simulink model "PLL_voltagesag"  (R2025a)
settings: Solver=FixedStepAuto  StartTime=0.0  StopTime=1  FixedStep=Ts  RelTol=1e-3
values from neighbouring files (symbols this model uses):
  C_dc = 2.25    [PLLpara.m]
  Cf1 = 0.01    [PLLpara.m]
  Cf2 = 0.01    [PLLpara.m]
  dt_sag = t_c    [GFMPara.m]    (also in GFMPara_exp.m; PLLpara.m; VFMPara.m; VFMPara_exp.m)
  f_switching = 20e3    (= 20000)    [GFMPara_exp.m]    (also in PLLpara.m = 10000; VFMPara_exp.m)
  Id0 = Id    [PLLpara.m]
  Iq01 = 0    [PLLpara.m]
  Iq02 = (Ug*cos(asin((Xg*Id+Rg*Iq)/Ug))+Id*Rg-Iq*Xg)*Cf2+Iq    [PLLpara.m]
  ki_pll1 = ki    [PLLpara.m]
  kp_pll1 = kp    [PLLpara.m]
  Lc = 1e-9    (= 1e-09)    [GFMPara.m]    (also in GFMPara_exp.m; PLLpara.m; VFMPara.m; VFMPara_exp.m)
  Lf = 0.0592    [GFMPara.m]    (also in GFMPara_exp.m; PLLpara.m = 0.05; VFMPara.m = 0.05; VFMPara_exp.m = 0.05)
  Lg1 = X1    [PLLpara.m]    (also in VFMPara.m; VFMPara_exp.m)
  Lgg = Xgg    [PLLpara.m]    (also in VFMPara.m; VFMPara_exp.m)
  Rf = 1e-3    (= 0.001)    [PLLpara.m]
  Rg1 = R1    [PLLpara.m]    (also in VFMPara.m; VFMPara_exp.m = 4*R1/5)
  Rgg = Rgg    [PLLpara.m]    (also in VFMPara.m; VFMPara_exp.m)
  Sbase = 1    [GFMPara.m]    (also in GFMPara_exp.m; PLLpara.m; VFMPara.m; VFMPara_exp.m)
  t0 = t_sim_start +t_start    [PLLpara.m]    (also in VFMPara_exp.m)
  t0_sag = t_sim_start +t_start    [GFMPara.m]    (also in GFMPara_exp.m; PLLpara.m = 20; VFMPara.m; VFMPara_exp.m = 20)
  Tc = 1/f_switching    (= 5e-05)    [GFMPara_exp.m]    (also in PLLpara.m = 0.0001; VFMPara_exp.m)
  tc = t_c    [PLLpara.m]    (also in VFMPara_exp.m)
  Ts = 1/Fs    (= 1e-05)    [GFMPara.m]    (also in GFMPara_exp.m = 1e-06; PLLpara.m = 1e-06; VFMPara.m = 5e-06; VFMPara_exp.m = 1e-06)
  v_sag = Ug_fault    [GFMPara.m]    (also in GFMPara_exp.m; PLLpara.m; VFMPara.m; VFMPara_exp.m)
  Vbase = 1    [GFMPara.m]    (also in GFMPara_exp.m; PLLpara.m; VFMPara.m; VFMPara_exp.m)
  Vdc = 2.5    [PLLpara.m]
  w_i_GFL1 = 1100 *2*pi    (= 6911.5038379)    [PLLpara.m]
  w_i_GFL2 = 1100 *2*pi    (= 6911.5038379)    [PLLpara.m]
  w_pll1 = 10 *2*pi    (= 62.8318530718)    [PLLpara.m]
  w_tau1 = 1500 *2*pi    (= 9424.77796077)    [PLLpara.m]
  Wbase = 2*pi*50    (= 314.159265359)    [GFMPara.m]    (also in GFMPara_exp.m; PLLpara.m; VFMPara.m; VFMPara_exp.m)
  Zbase = Vbase/Ibase    (= 1)    [GFMPara.m]    (also in GFMPara_exp.m; PLLpara.m; VFMPara.m; VFMPara_exp.m)
undefined symbols (not defined in the file or in its folder): DiscIntNeverNeededParam, dspblkCoreblockFVToolHelper, gcbh, initial, position, postfault_SEP, sigbuilder_block, w_max, w_min, Ws
libraries: spsVoltageMeasurementLib x80, spsCurrentMeasurementLib x75, spsIdealSwitchLib x30, spsThreePhaseSeriesRLCBranchLib x21, spsControlledVoltageSourceLib x18, spsSeriesRLCBranchLib x11, powerlib_extras x10, spsHalfBridgeConverterLib x6, spsThreePhaseBreakerLib x6, spsDCVoltageSourceLib x4, spsThreePhaseFaultLib x3, cstblocks x2
(part 1 of 5)
settings Model: Creator=admin_user  LastModifiedBy=yifan
settings SolverCC: AlgebraicLoopSolver=TrustRegion
settings DataIOCC: ReturnWorkspaceOutputs=off
settings ModelReferenceCC: EnableRefExpFcnMdlSchedulingChecks=on
settings RTWCC: GPUComputeCapability=3.5  DLArmComputeVersion=19.05

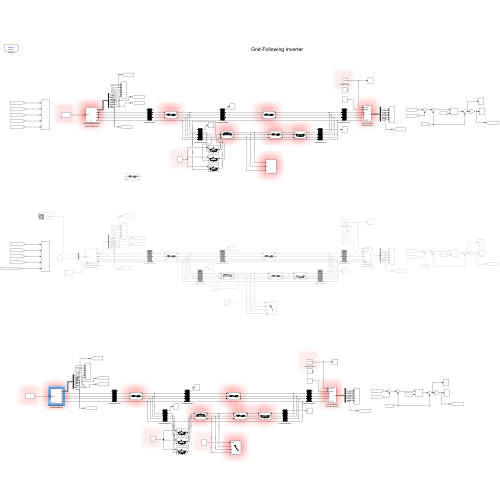
[thumbnail: Simulink's stored preview of the top-level diagram]
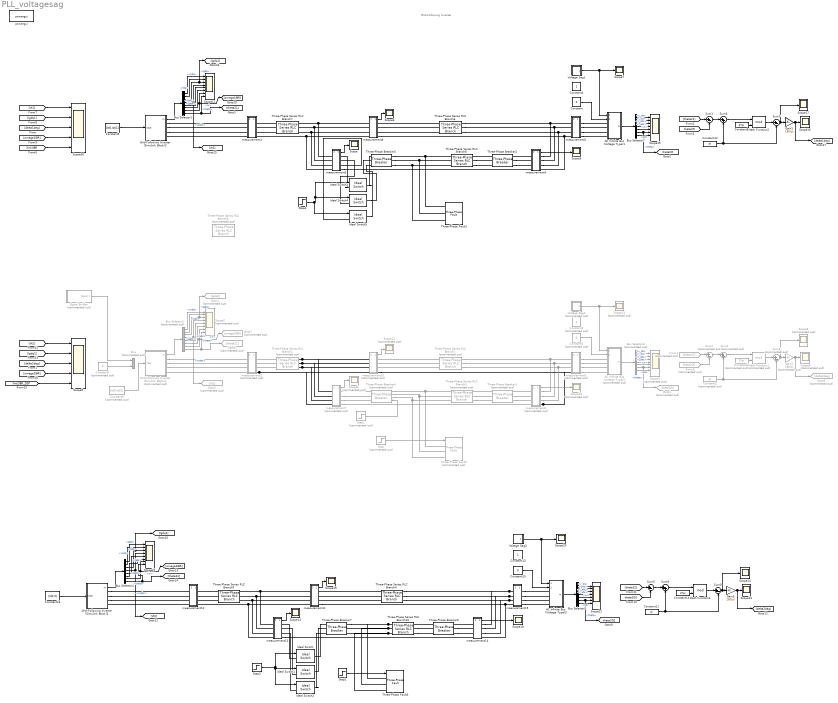
== system PLL_voltagesag ==
  note: Grid-Following Inverter
  AC Infinite Bus (Voltage Type)1 : Subsystem  AncestorBlock=|  mask{Ts=Ts, Sbase=Sbase, Vbase=Vbase, Wbase=Wbase, theta0=0, w=Wbase, R=1e-30}
      | SimplusGT/AC Infinite Bus
      | (Voltage Type)
      mask prompts: Ts "Ts (s), samping period"; Sbase "Sbase (VA), power base"; Vbase "Vbase (V), voltage base"; Wbase "Wbase (rad/s), frequency base"; theta0 "theta0 (rad), initial angle"; w "w (rad/s), frequency"; R "R (Ohm), resistance"
  AC Infinite Bus (Voltage Type)2 : Subsystem  Commented=on  AncestorBlock=|  mask{Ts=Ts, Sbase=Sbase, Vbase=Vbase, Wbase=Wbase, theta0=0, w=Wbase, R=1e-30}
      | SimplusGT/AC Infinite Bus
      | (Voltage Type)
      mask prompts: Ts "Ts (s), samping period"; Sbase "Sbase (VA), power base"; Vbase "Vbase (V), voltage base"; Wbase "Wbase (rad/s), frequency base"; theta0 "theta0 (rad), initial angle"; w "w (rad/s), frequency"; R "R (Ohm), resistance"
  AC Infinite Bus (Voltage Type)3 : Subsystem  AncestorBlock=|  mask{Ts=Ts, Sbase=Sbase, Vbase=Vbase, Wbase=Wbase, theta0=0, w=Wbase, R=1e-30}
      | SimplusGT/AC Infinite Bus
      | (Voltage Type)
      mask prompts: Ts "Ts (s), samping period"; Sbase "Sbase (VA), power base"; Vbase "Vbase (V), voltage base"; Wbase "Wbase (rad/s), frequency base"; theta0 "theta0 (rad), initial angle"; w "w (rad/s), frequency"; R "R (Ohm), resistance"
  Bus Selector1 : BusSelector  OutputSignals=vcdq,ildq,igdq,vcabc,ilabc,igabc,w,theta
  Bus Selector2 : BusSelector  Commented=on  OutputSignals=vcdq,ildq,igdq,vcabc,ilabc,igabc,w,theta
  Bus Selector3 : BusSelector  Commented=on  OutputSignals=v_dq,i_dq,v_abc,i_abc,w,theta,pq
  Bus Selector4 : BusSelector  OutputSignals=vcdq,ildq,igdq,vcabc,ilabc,igabc,w,theta
  Bus Selector5 : BusSelector  OutputSignals=v_dq,i_dq,v_abc,i_abc,w,theta,pq
  Bus Selector7 : BusSelector  OutputSignals=v_dq,i_dq,v_abc,i_abc,w,theta,pq
  Constant : Constant  Value=0
  Constant1 : Constant  Commented=on  Value=0
  Constant10 : Constant  Value=0
  Constant11 : Constant  Value=pi
  Constant12 : Constant  Value=pi
  Constant13 : Constant
  Constant14 : Constant  Value=2*pi
  Constant16 : Constant  Value=[Id0,0]
  Constant2 : Constant  Commented=on  Value=pi
  Constant3 : Constant  Commented=on
  Constant4 : Constant
  Constant5 : Constant  Value=[Id0,Iq01]
  Constant6 : Constant  Commented=on  Value=2*pi
  Constant7 : Constant  Commented=on  Value=0
  Constant8 : Constant  Commented=on  Value=[Id0,Iq02]
  Constant9 : Constant  Value=2*pi
  From4 : From  Commented=on  GotoTag=theta22
  From9 : From  Commented=on  GotoTag=theta2G2  TagVisibility=global
  Gain1 : Gain  Gain=180/pi
  Gain2 : Gain  Commented=on  Gain=180/pi
  Gain3 : Gain  Gain=180/pi
  Goto1 : Goto  Commented=on  GotoTag=theta2G2  TagVisibility=global
  Goto4 : Goto  Commented=on  GotoTag=Igdq2
  Goto5 : Goto  Commented=on  GotoTag=Vt2
  Goto6 : Goto  Commented=on  GotoTag=delta2deg
  Goto7 : Goto  Commented=on  GotoTag=omega2IBR
  Goto8 : Goto  Commented=on  GotoTag=theta22
  Grid-Following Inverter (Simulink Block)1 : Subsystem  Commented=on  AncestorBlock=|  mask{Ts=Ts, Sbase=Sbase, Vbase=Vbase, Wbase=Wbase, w_i=w_i_GFL2, w_pll=w_pll1, w_tau=w_tau1, Lf=Lf, Cf=Cf2, Lc=Lc}
      | SimplusGT/Grid-Following Inverter
      | (Simulink Block)
      mask prompts: Ts "Ts (s), sampling period"; Sbase "Sbase (VA), base power"; Vbase "Vbase (V), base voltage"; Wbase "Wbase (rad/s), base frequency"; w_i "w_i (rad/s), current-loop bandwidth"; w_pll "w_pll (rad/s), PLL bandwidth"; w_tau "w_tau (rad/s), PLL filter bandwidth"; Lf "Lf (pu), LCL filter"; Cf "Cf (pu), LCL filter"; Lc "Lc (pu), LCL filter"
  Grid-Following Inverter (Simulink Block)2 : Subsystem  AncestorBlock=|  mask{Ts=Ts, Sbase=Sbase, Vbase=Vbase, Wbase=Wbase, w_i=w_i_GFL1, w_pll=w_pll1, w_tau=w_tau1, Lf=Lf, Cf=Cf1, Lc=Lc}
      | SimplusGT/Grid-Following Inverter
      | (Simulink Block)
      mask prompts: Ts "Ts (s), sampling period"; Sbase "Sbase (VA), base power"; Vbase "Vbase (V), base voltage"; Wbase "Wbase (rad/s), base frequency"; w_i "w_i (rad/s), current-loop bandwidth"; w_pll "w_pll (rad/s), PLL bandwidth"; w_tau "w_tau (rad/s), PLL filter bandwidth"; Lf "Lf (pu), LCL filter"; Cf "Cf (pu), LCL filter"; Lc "Lc (pu), LCL filter"
  Grid-Following Inverter (Simulink Block)3 : Subsystem  AncestorBlock=|  mask{Ts=Ts, Sbase=Sbase, Vbase=Vbase, Wbase=Wbase, w_i=w_i_GFL2, w_pll=w_pll1, w_tau=w_tau1, Lf=Lf, Cf=Cf2, Lc=Lc}
      | SimplusGT/Grid-Following Inverter
      | (Simulink Block)
      mask prompts: Ts "Ts (s), sampling period"; Sbase "Sbase (VA), base power"; Vbase "Vbase (V), base voltage"; Wbase "Wbase (rad/s), base frequency"; w_i "w_i (rad/s), current-loop bandwidth"; w_pll "w_pll (rad/s), PLL bandwidth"; w_tau "w_tau (rad/s), PLL filter bandwidth"; Lf "Lf (pu), LCL filter"; Cf "Cf (pu), LCL filter"; Lc "Lc (pu), LCL filter"
  Ideal Switch{,1..5} (6 alike) : spsIdealSwitchLib/Ideal Switch  Ron=0.001  Lon=0  IC=0  Rs=5  Cs=1e-2  Measurements=off
  Math Function1 : Math  Commented=on  Operator=mod  SignedPower=on
  Math Function2 : Math  Operator=mod  SignedPower=on
  Math Function3 : Math  Operator=mod  SignedPower=on
  Mux : Mux  Commented=on  Inputs=2
  Scope{,5..7,14,16..20,23..24} (12 alike) : Scope
      Scope settings: ActiveDisplayYMinimum=-1.51038  ActiveDisplayYMaximum=1.38351
      Scope14 settings: ActiveDisplayYMinimum=-1.35141  ActiveDisplayYMaximum=1.22161
      Scope16 settings: ActiveDisplayYMinimum=-224.72735  ActiveDisplayYMaximum=224.86411  DataLoggingDecimation=10  DataLoggingVariableName=ScopeData6
      Scope17 settings: ActiveDisplayYMinimum=-3.92346  ActiveDisplayYMaximum=3.9238  DataLoggingDecimation=10  DataLoggingVariableName=log_Delta
      Scope18 settings: ActiveDisplayYMinimum=-0.66277  ActiveDisplayYMaximum=0.79991  DataLoggingVariableName=ScopeData2
      Scope19 settings: ActiveDisplayYMinimum=-3.26758  ActiveDisplayYMaximum=3.40018  DataLoggingVariableName=ScopeData3
      Scope20 settings: ActiveDisplayYMinimum=0.10658  ActiveDisplayYMaximum=1.05549  DataLoggingVariableName=ScopeData4
      Scope23 settings: ActiveDisplayYMinimum=-224.72735  ActiveDisplayYMaximum=224.86411  DataLoggingDecimation=10  DataLoggingVariableName=ScopeData7
      Scope24 settings: ActiveDisplayYMinimum=-3.92678  ActiveDisplayYMaximum=3.92693  DataLoggingDecimation=10  DataLoggingVariableName=log_Delta2
      Scope5 settings: ActiveDisplayYMinimum=-6.53351  ActiveDisplayYMaximum=8.12515  DataLoggingVariableName=ScopeData2
      Scope6 settings: ActiveDisplayYMinimum=-3.26758  ActiveDisplayYMaximum=3.40018  DataLoggingVariableName=ScopeData3
      Scope7 settings: ActiveDisplayYMinimum=0.10658  ActiveDisplayYMaximum=1.05549
  Scope{1,4,8,10,12..13} (6 alike) : Scope  Commented=on
      Scope1 settings: ActiveDisplayYMinimum=-4.56603  ActiveDisplayYMaximum=4.9186
      Scope10 settings: ActiveDisplayYMinimum=-0.66277  ActiveDisplayYMaximum=0.79991  DataLoggingVariableName=ScopeData2
      Scope12 settings: ActiveDisplayYMinimum=-3.26758  ActiveDisplayYMaximum=3.40018  DataLoggingVariableName=ScopeData3
      Scope13 settings: ActiveDisplayYMinimum=0.10658  ActiveDisplayYMaximum=1.05549  DataLoggingVariableName=ScopeData4
      Scope4 settings: ActiveDisplayYMinimum=-224.72735  ActiveDisplayYMaximum=224.86411  DataLoggingDecimation=10  DataLoggingVariableName=ScopeData7
      Scope8 settings: ActiveDisplayYMinimum=-3.92678  ActiveDisplayYMaximum=3.92693  DataLoggingDecimation=10  DataLoggingVariableName=log_Delta2
  Scope{11,15,21..22} (4 alike) : Scope  NumInputPorts=8
      Scope11 settings: ActiveDisplayYMinimum=-1.9339360338596787  ActiveDisplayYMaximum=2.6966948236171153  DataLoggingDecimation=10  DataLoggingVariableName=ScopeData3
      Scope15 settings: ActiveDisplayYMinimum=-0.125  ActiveDisplayYMaximum=1.125  DataLoggingVariableName=ScopeData5
      Scope21 settings: ActiveDisplayYMinimum=-3.066965643945478  ActiveDisplayYMaximum=2.9929362486112421  DataLoggingDecimation=10  DataLoggingVariableName=ScopeData5
      Scope22 settings: ActiveDisplayYMinimum=-0.125  ActiveDisplayYMaximum=1.125  DataLoggingVariableName=ScopeData6
  Scope2 : Scope  Commented=on  NumInputPorts=8
      settings: ActiveDisplayYMinimum=-2.4523  ActiveDisplayYMaximum=2.43362  DataLoggingDecimation=10  DataLoggingVariableName=ScopeData5
  Scope3 : Scope  Commented=on  NumInputPorts=8
      settings: ActiveDisplayYMinimum=-0.125  ActiveDisplayYMaximum=1.125  DataLoggingVariableName=ScopeData6
  Scope30 : Scope  NumInputPorts=5
      settings: TimeSpan=1  ActiveDisplayYMinimum=-2.69435  ActiveDisplayYMaximum=2.94504  DataLoggingDecimation=10
  Scope9 : Scope  NumInputPorts=5
      settings: TimeSpan=1  ActiveDisplayYMinimum=-2.46385  ActiveDisplayYMaximum=1.98854  DataLoggingDecimation=10  DataLoggingVariableName=ScopeData2
  Signal Builder : Subsystem  Tag=STV Subsys  Commented=on  LoadFcn=sigbuilder_block('load');  StartFcn=sigbuilder_block('start');  StopFcn=sigbuilder_block('stop');  ClipboardFcn=sigbuilder_block('clipboard');  mask(Sigbuilder block){tuvar=[0:10]}
      mask help: Simulink:masks:SigbuilderBlock_MD
      mask init:
      | if ~strcmp(get_param(bdroot(gcbh),'SimulationStatus'),'stopped') tuvar = sigbuilder_block('maskInit'); end
      settings: CopyFcn=sigbuilder_block('copy');  DeleteFcn=sigbuilder_block('delete');  ModelCloseFcn=sigbuilder_block('modelClose');  PreSaveFcn=sigbuilder_block('preSave');  PauseFcn=sigbuilder_block('pause');  ContinueFcn=sigbuilder_block('continue');  NameChangeFcn=sigbuilder_block('namechange');  OpenFcn=sigbuilder_block('open',[437.6 199.2 550.4 400 ]);  CloseFcn=sigbuilder_block('close');
      mask Display: plot(0, 0, 100, 100,[2, 2, 32, 32, 2], [68, 8, 8, 68, 68],[32, 2], [38, 38], [32, 19, 2],[53, 60, 44], [32, 17, 17, 2],[16, 16, 31, 31]);txt = getActiveGroup(gcbh);text(2, 100, txt,'verticalAlignment', 'top');
  Step : Step  Commented=on  Time=t0  SampleTime=0
  Step1 : Step  Commented=on  Time=t0+tc  Before=1  After=0  SampleTime=0
  Step2 : Step  Time=t0  SampleTime=0
  Step3 : Step  Time=t0+tc  Before=1  After=0  SampleTime=0
  Step4 : Step  Time=t0+tc  Before=1  After=0  SampleTime=0
  Sum{1,5,7,9} (4 alike) : Sum  Inputs=|+-
  Sum2 : Sum  Commented=on  Inputs=|+-
  Sum3 : Sum  Commented=on  Inputs=|++
  Sum4 : Sum  Commented=on  Inputs=|+-
  Sum6 : Sum  Inputs=|++
  Sum8 : Sum  Inputs=|++
  Three-Phase Series RLC Branch1 : spsThreePhaseSeriesRLCBranchLib/Three-Phase Series RLC Branch  Commented=on  LConnTagsString=A|B|C  RConnTagsString=A|B|C  BranchType=RL  Resistance=Rgg*Zbase  Inductance=Lgg*Zbase/Wbase  Capacitance=1/Wbase  Measurements=None
  Three-Phase Series RLC Branch{4,6,8,10} (4 alike) : spsThreePhaseSeriesRLCBranchLib/Three-Phase Series RLC Branch  LConnTagsString=A|B|C  RConnTagsString=A|B|C  BranchType=RL  Resistance=Rgg*Zbase  Inductance=Lgg*Zbase/Wbase  Capacitance=1/Wbase  Measurements=None
  Three-Phase Series RLC Branch2 : spsThreePhaseSeriesRLCBranchLib/Three-Phase Series RLC Branch  Commented=on  LConnTagsString=A|B|C  RConnTagsString=A|B|C  BranchType=RL  Resistance=Rg1*Zbase  Inductance=Lg1*Zbase/Wbase  Capacitance=1/Wbase  Measurements=None
  Three-Phase Series RLC Branch3 : spsThreePhaseSeriesRLCBranchLib/Three-Phase Series RLC Branch  Commented=on  LConnTagsString=A|B|C  RConnTagsString=A|B|C  BranchType=RL  Resistance=Rgg*Zbase  Inductance=Lgg*Zbase/Wbase  Capacitance=1/Wbase  Measurements=None
  Three-Phase Series RLC Branch5 : spsThreePhaseSeriesRLCBranchLib/Three-Phase Series RLC Branch  Commented=on  LConnTagsString=A|B|C  RConnTagsString=A|B|C  BranchType=RL  Resistance=1e-3 %Rgg*Zbase*(1-position)  Inductance=Lgg*Zbase/Wbase*0.1  Capacitance=1/Wbase  Measurements=None
  Three-Phase Series RLC Branch7 : spsThreePhaseSeriesRLCBranchLib/Three-Phase Series RLC Branch  LConnTagsString=A|B|C  RConnTagsString=A|B|C  BranchType=RL  Resistance=Rg1*Zbase  Inductance=Lg1*Zbase/Wbase  Capacitance=1/Wbase  Measurements=None
  Three-Phase Series RLC Branch9 : spsThreePhaseSeriesRLCBranchLib/Three-Phase Series RLC Branch  LConnTagsString=A|B|C  RConnTagsString=A|B|C  BranchType=RL  Resistance=Rg1*Zbase  Inductance=Lg1*Zbase/Wbase  Capacitance=1/Wbase  Measurements=None
  Three-Phase Breaker1 : spsThreePhaseBreakerLib/Three-Phase Breaker  Commented=on  InitialState=closed  SwitchA=on  SwitchB=on  SwitchC=on  SwitchTimes=[t0+tc]  External=off  BreakerResistance=0.01e-3  SnubberResistance=1e6  SnubberCapacitance=inf  Measurements=Breaker currents
  Three-Phase Breaker2 : spsThreePhaseBreakerLib/Three-Phase Breaker  InitialState=closed  SwitchA=on  SwitchB=on  SwitchC=on  SwitchTimes=[t0+tc]  External=off  BreakerResistance=0.01e-3  SnubberResistance=1e6  SnubberCapacitance=inf  Measurements=Breaker currents
  Three-Phase Breaker3 : spsThreePhaseBreakerLib/Three-Phase Breaker  InitialState=closed  SwitchA=on  SwitchB=on  SwitchC=on  SwitchTimes=[t0+tc]  External=off  BreakerResistance=0.1e-3  SnubberResistance=1e6  SnubberCapacitance=inf  Measurements=Breaker currents
  Three-Phase Breaker4 : spsThreePhaseBreakerLib/Three-Phase Breaker  Commented=on  InitialState=closed  SwitchA=on  SwitchB=on  SwitchC=on  SwitchTimes=[t0+tc]  External=on  BreakerResistance=0.1e-3  SnubberResistance=1e6  SnubberCapacitance=inf  Measurements=Breaker currents
  Three-Phase Breaker5 : spsThreePhaseBreakerLib/Three-Phase Breaker  InitialState=closed  SwitchA=on  SwitchB=on  SwitchC=on  SwitchTimes=[t0+tc]  External=off  BreakerResistance=0.01e-3  SnubberResistance=1e6  SnubberCapacitance=inf  Measurements=Breaker currents
  Three-Phase Breaker7 : spsThreePhaseBreakerLib/Three-Phase Breaker  InitialState=closed  SwitchA=on  SwitchB=on  SwitchC=on  SwitchTimes=[t0+tc]  External=off  BreakerResistance=0.1e-3  SnubberResistance=1e6  SnubberCapacitance=inf  Measurements=Breaker currents
  Three-Phase Fault1 : spsThreePhaseFaultLib/Three-Phase Fault  InitialStates=0  FaultA=on  FaultB=on  FaultC=on  GroundFault=on  SwitchTimes=[t0]  External=off  SwitchStatus=NaN  FaultResistance=Rf*Zbase  GroundResistance=0.01e-6  SnubberResistance=10e6  SnubberCapacitance=inf  Measurements=None
  Three-Phase Fault2 : spsThreePhaseFaultLib/Three-Phase Fault  Commented=on  InitialStates=0  FaultA=on  FaultB=on  FaultC=on  GroundFault=off  SwitchTimes=[t0]  External=on  SwitchStatus=NaN  FaultResistance=Rf*Zbase  GroundResistance=0.01e-6  SnubberResistance=10e6  SnubberCapacitance=inf  Measurements=None
  Three-Phase Fault3 : spsThreePhaseFaultLib/Three-Phase Fault  InitialStates=0  FaultA=on  FaultB=on  FaultC=on  GroundFault=on  SwitchTimes=[t0]  External=on  SwitchStatus=NaN  FaultResistance=Rf*Zbase  GroundResistance=0.01e-6  SnubberResistance=10e6  SnubberCapacitance=inf  Measurements=None
  Voltage Sag1 : Subsystem  AncestorBlock=SimplusGT/Single Pulse  mask{t0=t0_sag, dt=dt_sag, Am=v_sag}
      mask prompts: t0 "t0 (s), starting time"; dt "dt (s), pulse width"; Am "Am, pulse amplitude"
  Voltage Sag2 : Subsystem  Commented=on  AncestorBlock=SimplusGT/Single Pulse  mask{t0=t0_sag, dt=dt_sag, Am=v_sag}
      mask prompts: t0 "t0 (s), starting time"; dt "dt (s), pulse width"; Am "Am, pulse amplitude"
  Voltage Sag3 : Subsystem  AncestorBlock=SimplusGT/Single Pulse  mask{t0=t0_sag, dt=dt_sag, Am=v_sag}
      mask prompts: t0 "t0 (s), starting time"; dt "dt (s), pulse width"; Am "Am, pulse amplitude"
  measurement1 : Subsystem
      settings: PortSchema="{\"entries\":[{\"content\":{\"sides\":[{\"content\":{\"connectorIds\":[\"Out2\",\"LConn1\",\"LConn2\",\"LConn3\",\"LConn4\"]},\"type\":\"ConnectorPlacement.EquallySpacedRectSide\",\"uuid\":\"b97639c7-89ad-4c11-8fcc-ddc4f61f4533\"},{\"content\":{\"connectorIds\":[\"Out1\",\"RConn1\",\"RConn2\",\"RConn3\",\"RConn4\"],\"side\":\"RIGHT\"},\"type\":\"ConnectorPlacement.EquallySpacedRectSide\",\"uuid\":\"3b8f0759-83d7-4d3a-a5c5-bdf29e7cbe5b\"},{\"content\":{\"connectorIds\":[],\"side\":\"TOP\"},\"type\":\"ConnectorPlacement.EquallySpacedRectSide\",\"uuid\":\"1e391932-f1e1-4127-bfe0-28b7de5de667\"},{\"content\":{\"connectorIds\":[],\"side\":\"BOTTOM\"},\"type\":\"ConnectorPlacement.EquallySpacedRectSide\",\"uuid\":\"f0c236e9-048a-4270-a45f-ff2fecf0ec8b\"}]},\"type\":\"ConnectorPlacement.EquallySpacedConnector\",\"uuid\":\"002609f8-6c16-431f-ae58-b6d94c927972\"}],\"packageUris\":[\"http://schema.mathworks.com/mf0/Connector/R2020b\"],\"version\":\"1.0\"}"
  measurement10 : Subsystem  Commented=on
      settings: PortSchema="{\"entries\":[{\"content\":{\"sides\":[{\"content\":{\"connectorIds\":[\"Out2\",\"LConn1\",\"LConn2\",\"LConn3\",\"LConn4\"]},\"type\":\"ConnectorPlacement.EquallySpacedRectSide\",\"uuid\":\"b97639c7-89ad-4c11-8fcc-ddc4f61f4533\"},{\"content\":{\"connectorIds\":[\"Out1\",\"RConn1\",\"RConn2\",\"RConn3\",\"RConn4\"],\"side\":\"RIGHT\"},\"type\":\"ConnectorPlacement.EquallySpacedRectSide\",\"uuid\":\"3b8f0759-83d7-4d3a-a5c5-bdf29e7cbe5b\"},{\"content\":{\"connectorIds\":[],\"side\":\"TOP\"},\"type\":\"ConnectorPlacement.EquallySpacedRectSide\",\"uuid\":\"1e391932-f1e1-4127-bfe0-28b7de5de667\"},{\"content\":{\"connectorIds\":[],\"side\":\"BOTTOM\"},\"type\":\"ConnectorPlacement.EquallySpacedRectSide\",\"uuid\":\"f0c236e9-048a-4270-a45f-ff2fecf0ec8b\"}]},\"type\":\"ConnectorPlacement.EquallySpacedConnector\",\"uuid\":\"002609f8-6c16-431f-ae58-b6d94c927972\"}],\"packageUris\":[\"http://schema.mathworks.com/mf0/Connector/R2020b\"],\"version\":\"1.0\"}"
  measurement11 : Subsystem
      settings: PortSchema="{\"entries\":[{\"content\":{\"sides\":[{\"content\":{\"connectorIds\":[\"Out2\",\"LConn1\",\"LConn2\",\"LConn3\",\"LConn4\"]},\"type\":\"ConnectorPlacement.EquallySpacedRectSide\",\"uuid\":\"b97639c7-89ad-4c11-8fcc-ddc4f61f4533\"},{\"content\":{\"connectorIds\":[\"Out1\",\"RConn1\",\"RConn2\",\"RConn3\",\"RConn4\"],\"side\":\"RIGHT\"},\"type\":\"ConnectorPlacement.EquallySpacedRectSide\",\"uuid\":\"3b8f0759-83d7-4d3a-a5c5-bdf29e7cbe5b\"},{\"content\":{\"connectorIds\":[],\"side\":\"TOP\"},\"type\":\"ConnectorPlacement.EquallySpacedRectSide\",\"uuid\":\"1e391932-f1e1-4127-bfe0-28b7de5de667\"},{\"content\":{\"connectorIds\":[],\"side\":\"BOTTOM\"},\"type\":\"ConnectorPlacement.EquallySpacedRectSide\",\"uuid\":\"f0c236e9-048a-4270-a45f-ff2fecf0ec8b\"}]},\"type\":\"ConnectorPlacement.EquallySpacedConnector\",\"uuid\":\"002609f8-6c16-431f-ae58-b6d94c927972\"}],\"packageUris\":[\"http://schema.mathworks.com/mf0/Connector/R2020b\"],\"version\":\"1.0\"}"
  measurement12 : Subsystem
      settings: PortSchema="{\"entries\":[{\"content\":{\"sides\":[{\"content\":{\"connectorIds\":[\"Out2\",\"LConn1\",\"LConn2\",\"LConn3\",\"LConn4\"]},\"type\":\"ConnectorPlacement.EquallySpacedRectSide\",\"uuid\":\"b97639c7-89ad-4c11-8fcc-ddc4f61f4533\"},{\"content\":{\"connectorIds\":[\"Out1\",\"RConn1\",\"RConn2\",\"RConn3\",\"RConn4\"],\"side\":\"RIGHT\"},\"type\":\"ConnectorPlacement.EquallySpacedRectSide\",\"uuid\":\"3b8f0759-83d7-4d3a-a5c5-bdf29e7cbe5b\"},{\"content\":{\"connectorIds\":[],\"side\":\"TOP\"},\"type\":\"ConnectorPlacement.EquallySpacedRectSide\",\"uuid\":\"1e391932-f1e1-4127-bfe0-28b7de5de667\"},{\"content\":{\"connectorIds\":[],\"side\":\"BOTTOM\"},\"type\":\"ConnectorPlacement.EquallySpacedRectSide\",\"uuid\":\"f0c236e9-048a-4270-a45f-ff2fecf0ec8b\"}]},\"type\":\"ConnectorPlacement.EquallySpacedConnector\",\"uuid\":\"002609f8-6c16-431f-ae58-b6d94c927972\"}],\"packageUris\":[\"http://schema.mathworks.com/mf0/Connector/R2020b\"],\"version\":\"1.0\"}"
  measurement13 : Subsystem
      settings: PortSchema="{\"entries\":[{\"content\":{\"sides\":[{\"content\":{\"connectorIds\":[\"Out2\",\"LConn1\",\"LConn2\",\"LConn3\",\"LConn4\"]},\"type\":\"ConnectorPlacement.EquallySpacedRectSide\",\"uuid\":\"b97639c7-89ad-4c11-8fcc-ddc4f61f4533\"},{\"content\":{\"connectorIds\":[\"Out1\",\"RConn1\",\"RConn2\",\"RConn3\",\"RConn4\"],\"side\":\"RIGHT\"},\"type\":\"ConnectorPlacement.EquallySpacedRectSide\",\"uuid\":\"3b8f0759-83d7-4d3a-a5c5-bdf29e7cbe5b\"},{\"content\":{\"connectorIds\":[],\"side\":\"TOP\"},\"type\":\"ConnectorPlacement.EquallySpacedRectSide\",\"uuid\":\"1e391932-f1e1-4127-bfe0-28b7de5de667\"},{\"content\":{\"connectorIds\":[],\"side\":\"BOTTOM\"},\"type\":\"ConnectorPlacement.EquallySpacedRectSide\",\"uuid\":\"f0c236e9-048a-4270-a45f-ff2fecf0ec8b\"}]},\"type\":\"ConnectorPlacement.EquallySpacedConnector\",\"uuid\":\"002609f8-6c16-431f-ae58-b6d94c927972\"}],\"packageUris\":[\"http://schema.mathworks.com/mf0/Connector/R2020b\"],\"version\":\"1.0\"}"
  measurement14 : Subsystem
      settings: PortSchema="{\"entries\":[{\"content\":{\"sides\":[{\"content\":{\"connectorIds\":[\"Out2\",\"LConn1\",\"LConn2\",\"LConn3\",\"LConn4\"]},\"type\":\"ConnectorPlacement.EquallySpacedRectSide\",\"uuid\":\"b97639c7-89ad-4c11-8fcc-ddc4f61f4533\"},{\"content\":{\"connectorIds\":[\"Out1\",\"RConn1\",\"RConn2\",\"RConn3\",\"RConn4\"],\"side\":\"RIGHT\"},\"type\":\"ConnectorPlacement.EquallySpacedRectSide\",\"uuid\":\"3b8f0759-83d7-4d3a-a5c5-bdf29e7cbe5b\"},{\"content\":{\"connectorIds\":[],\"side\":\"TOP\"},\"type\":\"ConnectorPlacement.EquallySpacedRectSide\",\"uuid\":\"1e391932-f1e1-4127-bfe0-28b7de5de667\"},{\"content\":{\"connectorIds\":[],\"side\":\"BOTTOM\"},\"type\":\"ConnectorPlacement.EquallySpacedRectSide\",\"uuid\":\"f0c236e9-048a-4270-a45f-ff2fecf0ec8b\"}]},\"type\":\"ConnectorPlacement.EquallySpacedConnector\",\"uuid\":\"002609f8-6c16-431f-ae58-b6d94c927972\"}],\"packageUris\":[\"http://schema.mathworks.com/mf0/Connector/R2020b\"],\"version\":\"1.0\"}"
  measurement15 : Subsystem
      settings: PortSchema="{\"entries\":[{\"content\":{\"sides\":[{\"content\":{\"connectorIds\":[\"Out2\",\"LConn1\",\"LConn2\",\"LConn3\",\"LConn4\"]},\"type\":\"ConnectorPlacement.EquallySpacedRectSide\",\"uuid\":\"b97639c7-89ad-4c11-8fcc-ddc4f61f4533\"},{\"content\":{\"connectorIds\":[\"Out1\",\"RConn1\",\"RConn2\",\"RConn3\",\"RConn4\"],\"side\":\"RIGHT\"},\"type\":\"ConnectorPlacement.EquallySpacedRectSide\",\"uuid\":\"3b8f0759-83d7-4d3a-a5c5-bdf29e7cbe5b\"},{\"content\":{\"connectorIds\":[],\"side\":\"TOP\"},\"type\":\"ConnectorPlacement.EquallySpacedRectSide\",\"uuid\":\"1e391932-f1e1-4127-bfe0-28b7de5de667\"},{\"content\":{\"connectorIds\":[],\"side\":\"BOTTOM\"},\"type\":\"ConnectorPlacement.EquallySpacedRectSide\",\"uuid\":\"f0c236e9-048a-4270-a45f-ff2fecf0ec8b\"}]},\"type\":\"ConnectorPlacement.EquallySpacedConnector\",\"uuid\":\"002609f8-6c16-431f-ae58-b6d94c927972\"}],\"packageUris\":[\"http://schema.mathworks.com/mf0/Connector/R2020b\"],\"version\":\"1.0\"}"
  measurement2 : Subsystem  Commented=on
      settings: PortSchema="{\"entries\":[{\"content\":{\"sides\":[{\"content\":{\"connectorIds\":[\"Out2\",\"LConn1\",\"LConn2\",\"LConn3\",\"LConn4\"]},\"type\":\"ConnectorPlacement.EquallySpacedRectSide\",\"uuid\":\"b97639c7-89ad-4c11-8fcc-ddc4f61f4533\"},{\"content\":{\"connectorIds\":[\"Out1\",\"RConn1\",\"RConn2\",\"RConn3\",\"RConn4\"],\"side\":\"RIGHT\"},\"type\":\"ConnectorPlacement.EquallySpacedRectSide\",\"uuid\":\"3b8f0759-83d7-4d3a-a5c5-bdf29e7cbe5b\"},{\"content\":{\"connectorIds\":[],\"side\":\"TOP\"},\"type\":\"ConnectorPlacement.EquallySpacedRectSide\",\"uuid\":\"1e391932-f1e1-4127-bfe0-28b7de5de667\"},{\"content\":{\"connectorIds\":[],\"side\":\"BOTTOM\"},\"type\":\"ConnectorPlacement.EquallySpacedRectSide\",\"uuid\":\"f0c236e9-048a-4270-a45f-ff2fecf0ec8b\"}]},\"type\":\"ConnectorPlacement.EquallySpacedConnector\",\"uuid\":\"002609f8-6c16-431f-ae58-b6d94c927972\"}],\"packageUris\":[\"http://schema.mathworks.com/mf0/Connector/R2020b\"],\"version\":\"1.0\"}"
  measurement3 : Subsystem
      settings: PortSchema="{\"entries\":[{\"content\":{\"sides\":[{\"content\":{\"connectorIds\":[\"Out2\",\"LConn1\",\"LConn2\",\"LConn3\",\"LConn4\"]},\"type\":\"ConnectorPlacement.EquallySpacedRectSide\",\"uuid\":\"b97639c7-89ad-4c11-8fcc-ddc4f61f4533\"},{\"content\":{\"connectorIds\":[\"Out1\",\"RConn1\",\"RConn2\",\"RConn3\",\"RConn4\"],\"side\":\"RIGHT\"},\"type\":\"ConnectorPlacement.EquallySpacedRectSide\",\"uuid\":\"3b8f0759-83d7-4d3a-a5c5-bdf29e7cbe5b\"},{\"content\":{\"connectorIds\":[],\"side\":\"TOP\"},\"type\":\"ConnectorPlacement.EquallySpacedRectSide\",\"uuid\":\"1e391932-f1e1-4127-bfe0-28b7de5de667\"},{\"content\":{\"connectorIds\":[],\"side\":\"BOTTOM\"},\"type\":\"ConnectorPlacement.EquallySpacedRectSide\",\"uuid\":\"f0c236e9-048a-4270-a45f-ff2fecf0ec8b\"}]},\"type\":\"ConnectorPlacement.EquallySpacedConnector\",\"uuid\":\"002609f8-6c16-431f-ae58-b6d94c927972\"}],\"packageUris\":[\"http://schema.mathworks.com/mf0/Connector/R2020b\"],\"version\":\"1.0\"}"
  measurement4 : Subsystem
      settings: PortSchema="{\"entries\":[{\"content\":{\"sides\":[{\"content\":{\"connectorIds\":[\"Out2\",\"LConn1\",\"LConn2\",\"LConn3\",\"LConn4\"]},\"type\":\"ConnectorPlacement.EquallySpacedRectSide\",\"uuid\":\"b97639c7-89ad-4c11-8fcc-ddc4f61f4533\"},{\"content\":{\"connectorIds\":[\"Out1\",\"RConn1\",\"RConn2\",\"RConn3\",\"RConn4\"],\"side\":\"RIGHT\"},\"type\":\"ConnectorPlacement.EquallySpacedRectSide\",\"uuid\":\"3b8f0759-83d7-4d3a-a5c5-bdf29e7cbe5b\"},{\"content\":{\"connectorIds\":[],\"side\":\"TOP\"},\"type\":\"ConnectorPlacement.EquallySpacedRectSide\",\"uuid\":\"1e391932-f1e1-4127-bfe0-28b7de5de667\"},{\"content\":{\"connectorIds\":[],\"side\":\"BOTTOM\"},\"type\":\"ConnectorPlacement.EquallySpacedRectSide\",\"uuid\":\"f0c236e9-048a-4270-a45f-ff2fecf0ec8b\"}]},\"type\":\"ConnectorPlacement.EquallySpacedConnector\",\"uuid\":\"002609f8-6c16-431f-ae58-b6d94c927972\"}],\"packageUris\":[\"http://schema.mathworks.com/mf0/Connector/R2020b\"],\"version\":\"1.0\"}"
  measurement5 : Subsystem
      settings: PortSchema="{\"entries\":[{\"content\":{\"sides\":[{\"content\":{\"connectorIds\":[\"Out2\",\"LConn1\",\"LConn2\",\"LConn3\",\"LConn4\"]},\"type\":\"ConnectorPlacement.EquallySpacedRectSide\",\"uuid\":\"b97639c7-89ad-4c11-8fcc-ddc4f61f4533\"},{\"content\":{\"connectorIds\":[\"Out1\",\"RConn1\",\"RConn2\",\"RConn3\",\"RConn4\"],\"side\":\"RIGHT\"},\"type\":\"ConnectorPlacement.EquallySpacedRectSide\",\"uuid\":\"3b8f0759-83d7-4d3a-a5c5-bdf29e7cbe5b\"},{\"content\":{\"connectorIds\":[],\"side\":\"TOP\"},\"type\":\"ConnectorPlacement.EquallySpacedRectSide\",\"uuid\":\"1e391932-f1e1-4127-bfe0-28b7de5de667\"},{\"content\":{\"connectorIds\":[],\"side\":\"BOTTOM\"},\"type\":\"ConnectorPlacement.EquallySpacedRectSide\",\"uuid\":\"f0c236e9-048a-4270-a45f-ff2fecf0ec8b\"}]},\"type\":\"ConnectorPlacement.EquallySpacedConnector\",\"uuid\":\"002609f8-6c16-431f-ae58-b6d94c927972\"}],\"packageUris\":[\"http://schema.mathworks.com/mf0/Connector/R2020b\"],\"version\":\"1.0\"}"
  measurement6 : Subsystem
      settings: PortSchema="{\"entries\":[{\"content\":{\"sides\":[{\"content\":{\"connectorIds\":[\"Out2\",\"LConn1\",\"LConn2\",\"LConn3\",\"LConn4\"]},\"type\":\"ConnectorPlacement.EquallySpacedRectSide\",\"uuid\":\"b97639c7-89ad-4c11-8fcc-ddc4f61f4533\"},{\"content\":{\"connectorIds\":[\"Out1\",\"RConn1\",\"RConn2\",\"RConn3\",\"RConn4\"],\"side\":\"RIGHT\"},\"type\":\"ConnectorPlacement.EquallySpacedRectSide\",\"uuid\":\"3b8f0759-83d7-4d3a-a5c5-bdf29e7cbe5b\"},{\"content\":{\"connectorIds\":[],\"side\":\"TOP\"},\"type\":\"ConnectorPlacement.EquallySpacedRectSide\",\"uuid\":\"1e391932-f1e1-4127-bfe0-28b7de5de667\"},{\"content\":{\"connectorIds\":[],\"side\":\"BOTTOM\"},\"type\":\"ConnectorPlacement.EquallySpacedRectSide\",\"uuid\":\"f0c236e9-048a-4270-a45f-ff2fecf0ec8b\"}]},\"type\":\"ConnectorPlacement.EquallySpacedConnector\",\"uuid\":\"002609f8-6c16-431f-ae58-b6d94c927972\"}],\"packageUris\":[\"http://schema.mathworks.com/mf0/Connector/R2020b\"],\"version\":\"1.0\"}"
  measurement7 : Subsystem  Commented=on
      settings: PortSchema="{\"entries\":[{\"content\":{\"sides\":[{\"content\":{\"connectorIds\":[\"Out2\",\"LConn1\",\"LConn2\",\"LConn3\",\"LConn4\"]},\"type\":\"ConnectorPlacement.EquallySpacedRectSide\",\"uuid\":\"b97639c7-89ad-4c11-8fcc-ddc4f61f4533\"},{\"content\":{\"connectorIds\":[\"Out1\",\"RConn1\",\"RConn2\",\"RConn3\",\"RConn4\"],\"side\":\"RIGHT\"},\"type\":\"ConnectorPlacement.EquallySpacedRectSide\",\"uuid\":\"3b8f0759-83d7-4d3a-a5c5-bdf29e7cbe5b\"},{\"content\":{\"connectorIds\":[],\"side\":\"TOP\"},\"type\":\"ConnectorPlacement.EquallySpacedRectSide\",\"uuid\":\"1e391932-f1e1-4127-bfe0-28b7de5de667\"},{\"content\":{\"connectorIds\":[],\"side\":\"BOTTOM\"},\"type\":\"ConnectorPlacement.EquallySpacedRectSide\",\"uuid\":\"f0c236e9-048a-4270-a45f-ff2fecf0ec8b\"}]},\"type\":\"ConnectorPlacement.EquallySpacedConnector\",\"uuid\":\"002609f8-6c16-431f-ae58-b6d94c927972\"}],\"packageUris\":[\"http://schema.mathworks.com/mf0/Connector/R2020b\"],\"version\":\"1.0\"}"
  measurement8 : Subsystem  Commented=on
      settings: PortSchema="{\"entries\":[{\"content\":{\"sides\":[{\"content\":{\"connectorIds\":[\"Out2\",\"LConn1\",\"LConn2\",\"LConn3\",\"LConn4\"]},\"type\":\"ConnectorPlacement.EquallySpacedRectSide\",\"uuid\":\"b97639c7-89ad-4c11-8fcc-ddc4f61f4533\"},{\"content\":{\"connectorIds\":[\"Out1\",\"RConn1\",\"RConn2\",\"RConn3\",\"RConn4\"],\"side\":\"RIGHT\"},\"type\":\"ConnectorPlacement.EquallySpacedRectSide\",\"uuid\":\"3b8f0759-83d7-4d3a-a5c5-bdf29e7cbe5b\"},{\"content\":{\"connectorIds\":[],\"side\":\"TOP\"},\"type\":\"ConnectorPlacement.EquallySpacedRectSide\",\"uuid\":\"1e391932-f1e1-4127-bfe0-28b7de5de667\"},{\"content\":{\"connectorIds\":[],\"side\":\"BOTTOM\"},\"type\":\"ConnectorPlacement.EquallySpacedRectSide\",\"uuid\":\"f0c236e9-048a-4270-a45f-ff2fecf0ec8b\"}]},\"type\":\"ConnectorPlacement.EquallySpacedConnector\",\"uuid\":\"002609f8-6c16-431f-ae58-b6d94c927972\"}],\"packageUris\":[\"http://schema.mathworks.com/mf0/Connector/R2020b\"],\"version\":\"1.0\"}"
  measurement9 : Subsystem  Commented=on
      settings: PortSchema="{\"entries\":[{\"content\":{\"sides\":[{\"content\":{\"connectorIds\":[\"Out2\",\"LConn1\",\"LConn2\",\"LConn3\",\"LConn4\"]},\"type\":\"ConnectorPlacement.EquallySpacedRectSide\",\"uuid\":\"b97639c7-89ad-4c11-8fcc-ddc4f61f4533\"},{\"content\":{\"connectorIds\":[\"Out1\",\"RConn1\",\"RConn2\",\"RConn3\",\"RConn4\"],\"side\":\"RIGHT\"},\"type\":\"ConnectorPlacement.EquallySpacedRectSide\",\"uuid\":\"3b8f0759-83d7-4d3a-a5c5-bdf29e7cbe5b\"},{\"content\":{\"connectorIds\":[],\"side\":\"TOP\"},\"type\":\"ConnectorPlacement.EquallySpacedRectSide\",\"uuid\":\"1e391932-f1e1-4127-bfe0-28b7de5de667\"},{\"content\":{\"connectorIds\":[],\"side\":\"BOTTOM\"},\"type\":\"ConnectorPlacement.EquallySpacedRectSide\",\"uuid\":\"f0c236e9-048a-4270-a45f-ff2fecf0ec8b\"}]},\"type\":\"ConnectorPlacement.EquallySpacedConnector\",\"uuid\":\"002609f8-6c16-431f-ae58-b6d94c927972\"}],\"packageUris\":[\"http://schema.mathworks.com/mf0/Connector/R2020b\"],\"version\":\"1.0\"}"
  powergui : spspowerguiLib/powergui  Priority=1  SimulationMode=Discrete  SampleTime=Ts  frequency=60  Iterations=50  frequencyindice=0  Pbase=100e6  ErrMax=1e-4  UnitsV=kV  UnitsW=MW  buscounter=0  FunctionMessages=off  echomessages=off  EnableUseOfTLC=off  CurrentSourceSwitches=off  DisableSnubberDevices=off  DisableRonSwitches=off  DisableVfSwitches=off  DisplayEquations=off  AutomaticDiscreteSolvers=off  SolverType=Tustin/Backward Euler (TBE)  Interpol=off  ExternalGateDelay=off  methode=off  Ts=100  x0status=blocks  SPID=on  SwTol=0  HookPort=off  NonlinearTolerance=1e-4  nMaxIteration=100  ContinueOnMaxIteration=off  RestoreLinks=warning  ResistiveCurrentMeasurement=off  Frange=[0:2:500]  Ylog=off  Xlog=on  ShowGrid=off  save=off  variable=ZData  structure=0  ZoomFFT=off  StartTime=0.0  cycles=1  DisplayStyle=1  fundamental=60  FreqAxis=off  MaxFrequency=1000  frequencyindicesteady=1  RmsSteady=1  display=off
  tag scope: theta2G2=global, theta2G=global
  wires:
  [theta21] -> Sum1/1
  Bus Selector1/7 -> [omega1IBR], Scope11/7  "<w>"
  Grid-Following Inverter (Simulink Block)2/1(m) -> Bus Selector1/1
  Bus Selector1/2 -> Scope11/2  "<ildq>"
  Bus Selector1/5 -> Scope11/5  "<ilabc>"
  Constant12/1 -> Sum6/2, Sum7/2
  Sum1/1 -> Sum6/1
  Bus Selector7/3 -> Scope15/3  "<v_abc>"
  AC Infinite Bus (Voltage Type)1/1(m) -> Bus Selector7/1
  Constant9/1 -> Math Function2/2
  [theta2G] -> Sum1/2
  Gain1/1 -> [delta1deg], Scope16/1
  Bus Selector1/6 -> Scope11/6  "<igabc>"
  Bus Selector7/4 -> Scope15/4  "<i_abc>"
  Bus Selector7/5 -> Scope15/5  "<w>"
  Sum7/1 -> Scope17/1, Gain1/1
  Sum6/1 -> Math Function2/1
  Math Function2/1 -> Sum7/1
  Bus Selector7/7 -> Scope15/7  "<pq>"
  Bus Selector7/6 -> [theta2G], Scope15/6  "<theta>"
  Bus Selector7/1 -> Scope15/1  "<v_dq>"
  Bus Selector1/4 -> [Vt1], Scope11/4  "<vcabc>"
  Bus Selector1/1 -> Scope11/1  "<vcdq>"
  Bus Selector1/3 -> [Igdq1], Scope11/3  "<igdq>"
  Constant/1 -> AC Infinite Bus (Voltage Type)1/2(Phase)
  Bus Selector7/2 -> Scope15/2  "<i_dq>"
  Bus Selector1/8 -> [theta21], Scope11/8  "<theta>"
  [Vt1] -> Scope30/1
  [Igdq1] -> Scope30/2
  [Xint1IBR] -> Scope30/5
  [delta1deg] -> Scope30/3
  [omega1IBR] -> Scope30/4
  measurement3/1(Iabc) -> Scope/1
  measurement4/1(Iabc) -> Scope5/1
  measurement6/1(Iabc) -> Scope6/1
  Voltage Sag1/1(Out) -> Scope7/1, AC Infinite Bus (Voltage Type)1/1(v_mag)
  Constant6/1 -> Math Function1/2
  Bus Selector2/5 -> Scope2/5  "<ilabc>"
  Bus Selector3/2 -> Scope3/2  "<i_dq>"
  Gain2/1 -> Goto6/1, Scope4/1
  Bus Selector2/8 -> Goto8/1, Scope2/8  "<theta>"
  Constant2/1 -> Sum3/2, Sum4/2
  Bus Selector3/1 -> Scope3/1  "<v_dq>"
  Constant1/1 -> AC Infinite Bus (Voltage Type)2/2(Phase)
  Bus Selector2/3 -> Goto4/1, Scope2/3  "<igdq>"
  From9/1 -> Sum2/2
  [omega2IBR] -> Scope9/4
  Grid-Following Inverter (Simulink Block)1/1(m) -> Bus Selector2/1
  Voltage Sag2/1(Out) -> Scope13/1, AC Infinite Bus (Voltage Type)2/1(v_mag)
  Bus Selector2/1 -> Scope2/1  "<vcdq>"
  measurement7/1(Iabc) -> Scope1/1
  Bus Selector2/4 -> Goto5/1, Scope2/4  "<vcabc>"
  measurement10/1(Iabc) -> Scope12/1
  measurement8/1(Iabc) -> Scope10/1
  [Igdq2] -> Scope9/2
  [Vt2] -> Scope9/1
  [delta2deg] -> Scope9/3
  Bus Selector3/4 -> Scope3/4  "<i_abc>"
  Bus Selector3/7 -> Scope3/7  "<pq>"
  Sum2/1 -> Sum3/1
  Bus Selector2/2 -> Scope2/2  "<ildq>"
  Sum3/1 -> Math Function1/1
  Bus Selector3/6 -> Goto1/1, Scope3/6  "<theta>"
  Math Function1/1 -> Sum4/1
  Bus Selector2/7 -> Goto7/1, Scope2/7  "<w>"
  Bus Selector3/5 -> Scope3/5  "<w>"
  AC Infinite Bus (Voltage Type)2/1(m) -> Bus Selector3/1
  Bus Selector3/3 -> Scope3/3  "<v_abc>"
  From4/1 -> Sum2/1
  Sum4/1 -> Scope8/1, Gain2/1
  Bus Selector2/6 -> Scope2/6  "<igabc>"
  Constant7/1 -> Mux/2
  Signal Builder/1(Signal 1) -> Mux/1
  Constant5/1 -> Grid-Following Inverter (Simulink Block)2/1(ildq*)
  Constant8/1 -> Grid-Following Inverter (Simulink Block)1/1(ildq*)
  Step/1 -> Three-Phase Fault2/1
  Step1/1 -> Three-Phase Breaker4/1
  Step2/1 -> Three-Phase Fault3/1
  Math Function3/1 -> Sum9/1
  Bus Selector4/2 -> Scope21/2  "<ildq>"
  Bus Selector5/3 -> Scope22/3  "<v_abc>"
  Voltage Sag3/1(Out) -> Scope20/1, AC Infinite Bus (Voltage Type)3/1(v_mag)
  Grid-Following Inverter (Simulink Block)3/1(m) -> Bus Selector4/1
  Constant16/1 -> Grid-Following Inverter (Simulink Block)3/1(ildq*)
  Constant11/1 -> Sum8/2, Sum9/2
  measurement13/1(Iabc) -> Scope14/1
  Bus Selector4/8 -> [theta22], Scope21/8  "<theta>"
  Bus Selector4/6 -> Scope21/6  "<igabc>"
  Sum9/1 -> Scope24/1, Gain3/1
  [theta22] -> Sum5/1
  Sum5/1 -> Sum8/1
  AC Infinite Bus (Voltage Type)3/1(m) -> Bus Selector5/1
  [theta2G2] -> Sum5/2
  measurement14/1(Iabc) -> Scope18/1
  Bus Selector5/1 -> Scope22/1  "<v_dq>"
  Bus Selector5/5 -> Scope22/5  "<w>"
  Bus Selector4/7 -> [omega2IBR], Scope21/7  "<w>"
  Bus Selector4/5 -> Scope21/5  "<ilabc>"
  Bus Selector4/4 -> [Vt2], Scope21/4  "<vcabc>"
  Bus Selector4/3 -> [Igdq2], Scope21/3  "<igdq>"
  measurement11/1(Iabc) -> Scope19/1
  Constant10/1 -> AC Infinite Bus (Voltage Type)3/2(Phase)
  Bus Selector5/4 -> Scope22/4  "<i_abc>"
  Sum8/1 -> Math Function3/1
  Constant14/1 -> Math Function3/2
  Bus Selector5/2 -> Scope22/2  "<i_dq>"
  Gain3/1 -> [delta2deg], Scope23/1
  Bus Selector5/6 -> [theta2G2], Scope22/6  "<theta>"
  Bus Selector5/7 -> Scope22/7  "<pq>"
  Bus Selector4/1 -> Scope21/1  "<vcdq>"
  Step3/1 -> Ideal Switch/1, Ideal Switch2/1, Ideal Switch1/1
  Step4/1 -> Ideal Switch5/1, Ideal Switch4/1, Ideal Switch3/1
  [Xint2IBR_DSP] -> Scope9/5
  connections:
  Grid-Following Inverter (Simulink Block)2/RConn1 -- measurement1/LConn1
  Grid-Following Inverter (Simulink Block)2/RConn2 -- measurement1/LConn2
  Grid-Following Inverter (Simulink Block)2/RConn3 -- measurement1/LConn3
  measurement1/LConn4 -- Grid-Following Inverter (Simulink Block)2/RConn4
  measurement5/LConn4 -- measurement6/RConn4 -- measurement4/RConn4
  measurement5/RConn4 -- AC Infinite Bus (Voltage Type)1/LConn4
  measurement5/RConn1 -- AC Infinite Bus (Voltage Type)1/LConn1
  measurement5/RConn2 -- AC Infinite Bus (Voltage Type)1/LConn2
  measurement5/RConn3 -- AC Infinite Bus (Voltage Type)1/LConn3
  measurement4/RConn1 -- Three-Phase Series RLC Branch6/LConn1 -- measurement5/LConn1
  measurement4/RConn2 -- Three-Phase Series RLC Branch6/LConn2 -- measurement5/LConn2
  measurement4/RConn3 -- Three-Phase Series RLC Branch6/LConn3 -- measurement5/LConn3
  Three-Phase Series RLC Branch7/RConn3 -- measurement1/RConn3
  Three-Phase Series RLC Branch7/RConn2 -- measurement1/RConn2
  Three-Phase Series RLC Branch7/RConn1 -- measurement1/RConn1
  measurement6/LConn3 -- measurement3/LConn3 -- Three-Phase Series RLC Branch7/LConn3
  measurement6/LConn1 -- measurement3/LConn1 -- Three-Phase Series RLC Branch7/LConn1
  measurement6/LConn2 -- measurement3/LConn2 -- Three-Phase Series RLC Branch7/LConn2
  measurement3/RConn4 -- measurement4/LConn4
  measurement6/LConn4 -- measurement3/LConn4 -- measurement1/RConn4
  Three-Phase Fault1/LConn1 -- Three-Phase Breaker3/LConn3 -- Three-Phase Series RLC Branch8/RConn1
  Three-Phase Fault1/LConn2 -- Three-Phase Breaker3/LConn2 -- Three-Phase Series RLC Branch8/RConn2
  Three-Phase Fault1/LConn3 -- Three-Phase Breaker3/LConn1 -- Three-Phase Series RLC Branch8/RConn3
  Three-Phase Series RLC Branch6/RConn1 -- measurement6/RConn1
  Three-Phase Series RLC Branch6/RConn2 -- measurement6/RConn2
  Three-Phase Series RLC Branch6/RConn3 -- measurement6/RConn3
  measurement4/LConn1 -- Three-Phase Breaker2/RConn1
  Three-Phase Breaker2/LConn1 -- Three-Phase Series RLC Branch8/LConn1
  Three-Phase Series RLC Branch8/LConn2 -- Three-Phase Breaker2/LConn2
  Three-Phase Series RLC Branch8/LConn3 -- Three-Phase Breaker2/LConn3
  Three-Phase Breaker2/RConn3 -- measurement4/LConn3
  Three-Phase Breaker2/RConn2 -- measurement4/LConn2
  Three-Phase Series RLC Branch2/LConn1 -- measurement10/LConn1 -- measurement7/LConn1
  measurement8/RConn2 -- Three-Phase Series RLC Branch1/LConn2 -- measurement9/LConn2
  Three-Phase Series RLC Branch2/LConn2 -- measurement10/LConn2 -- measurement7/LConn2
  Three-Phase Fault2/LConn2 -- Three-Phase Breaker4/LConn2 -- Three-Phase Series RLC Branch3/RConn2
  measurement8/RConn4 -- measurement9/LConn4 -- measurement10/RConn4
  Three-Phase Series RLC Branch2/LConn3 -- measurement10/LConn3 -- measurement7/LConn3
  measurement8/RConn1 -- Three-Phase Series RLC Branch1/LConn1 -- measurement9/LConn1
  Three-Phase Fault2/LConn1 -- Three-Phase Breaker4/LConn3 -- Three-Phase Series RLC Branch3/RConn1
  Three-Phase Fault2/LConn3 -- Three-Phase Breaker4/LConn1 -- Three-Phase Series RLC Branch3/RConn3
  measurement2/RConn4 -- measurement10/LConn4 -- measurement7/LConn4
  measurement8/RConn3 -- Three-Phase Series RLC Branch1/LConn3 -- measurement9/LConn3
  measurement9/RConn3 -- AC Infinite Bus (Voltage Type)2/LConn3
  Three-Phase Series RLC Branch3/LConn2 -- Three-Phase Breaker1/LConn2
  measurement7/RConn4 -- measurement8/LConn4
  Three-Phase Series RLC Branch2/RConn2 -- measurement2/RConn2
  Grid-Following Inverter (Simulink Block)1/RConn2 -- measurement2/LConn2
  Three-Phase Series RLC Branch2/RConn1 -- measurement2/RConn1
  measurement2/LConn4 -- Grid-Following Inverter (Simulink Block)1/RConn4
  Three-Phase Series RLC Branch2/RConn3 -- measurement2/RConn3
  measurement9/RConn4 -- AC Infinite Bus (Voltage Type)2/LConn4
  Three-Phase Breaker4/RConn3 -- measurement7/RConn1
  Grid-Following Inverter (Simulink Block)1/RConn1 -- measurement2/LConn1
  measurement8/LConn1 -- Three-Phase Breaker1/RConn1
  measurement9/RConn1 -- AC Infinite Bus (Voltage Type)2/LConn1
  Three-Phase Series RLC Branch1/RConn2 -- measurement10/RConn2
  Grid-Following Inverter (Simulink Block)1/RConn3 -- measurement2/LConn3
  measurement9/RConn2 -- AC Infinite Bus (Voltage Type)2/LConn2
  Three-Phase Series RLC Branch1/RConn1 -- measurement10/RConn1
  Three-Phase Breaker1/RConn3 -- measurement8/LConn3
  Three-Phase Breaker1/RConn2 -- measurement8/LConn2
  Three-Phase Series RLC Branch1/RConn3 -- measurement10/RConn3
  Three-Phase Breaker1/LConn1 -- Three-Phase Series RLC Branch3/LConn1
  Three-Phase Series RLC Branch3/LConn3 -- Three-Phase Breaker1/LConn3
  measurement7/RConn2 -- Three-Phase Breaker4/RConn2
  measurement7/RConn3 -- Three-Phase Breaker4/RConn1
  measurement13/LConn3 -- measurement11/LConn3 -- Three-Phase Series RLC Branch9/LConn3
  Three-Phase Series RLC Branch10/RConn2 -- Three-Phase Breaker7/LConn2 -- Three-Phase Fault3/LConn2
  measurement15/LConn3 -- measurement14/RConn3 -- Three-Phase Series RLC Branch4/LConn3
  measurement13/LConn2 -- measurement11/LConn2 -- Three-Phase Series RLC Branch9/LConn2
  Three-Phase Series RLC Branch10/RConn3 -- Three-Phase Breaker7/LConn1 -- Three-Phase Fault3/LConn3
  measurement13/LConn1 -- measurement11/LConn1 -- Three-Phase Series RLC Branch9/LConn1
  Three-Phase Series RLC Branch10/RConn1 -- Three-Phase Breaker7/LConn3 -- Three-Phase Fault3/LConn1
  measurement11/RConn4 -- measurement15/LConn4 -- measurement14/RConn4
  measurement13/LConn4 -- measurement11/LConn4 -- measurement12/RConn4
  measurement15/LConn2 -- measurement14/RConn2 -- Three-Phase Series RLC Branch4/LConn2
  measurement15/LConn1 -- measurement14/RConn1 -- Three-Phase Series RLC Branch4/LConn1
  Three-Phase Series RLC Branch10/LConn3 -- Three-Phase Breaker5/LConn3
  Three-Phase Series RLC Branch4/RConn2 -- measurement11/RConn2
  measurement15/RConn1 -- AC Infinite Bus (Voltage Type)3/LConn1
  measurement15/RConn4 -- AC Infinite Bus (Voltage Type)3/LConn4
  measurement13/RConn4 -- measurement14/LConn4
  Three-Phase Breaker5/RConn2 -- measurement14/LConn2
  Three-Phase Breaker5/RConn3 -- measurement14/LConn3
  measurement14/LConn1 -- Three-Phase Breaker5/RConn1
  Three-Phase Series RLC Branch9/RConn1 -- measurement12/RConn1
  Three-Phase Series RLC Branch9/RConn2 -- measurement12/RConn2
  Three-Phase Series RLC Branch9/RConn3 -- measurement12/RConn3
  Three-Phase Series RLC Branch10/LConn2 -- Three-Phase Breaker5/LConn2
  Three-Phase Series RLC Branch4/RConn3 -- measurement11/RConn3
  measurement15/RConn2 -- AC Infinite Bus (Voltage Type)3/LConn2
  Grid-Following Inverter (Simulink Block)3/RConn2 -- measurement12/LConn2
  measurement15/RConn3 -- AC Infinite Bus (Voltage Type)3/LConn3
  Three-Phase Series RLC Branch4/RConn1 -- measurement11/RConn1
  Three-Phase Breaker5/LConn1 -- Three-Phase Series RLC Branch10/LConn1
  Grid-Following Inverter (Simulink Block)3/RConn3 -- measurement12/LConn3
  Grid-Following Inverter (Simulink Block)3/RConn1 -- measurement12/LConn1
  measurement12/LConn4 -- Grid-Following Inverter (Simulink Block)3/RConn4
  Ideal Switch/RConn1 -- Three-Phase Breaker7/RConn3
  Ideal Switch/LConn1 -- measurement13/RConn1
  Ideal Switch1/RConn1 -- Three-Phase Breaker7/RConn2
  Ideal Switch1/LConn1 -- measurement13/RConn2
  Ideal Switch2/RConn1 -- Three-Phase Breaker7/RConn1
  Ideal Switch2/LConn1 -- measurement13/RConn3
  Ideal Switch3/RConn1 -- Three-Phase Breaker3/RConn3
  Ideal Switch3/LConn1 -- measurement3/RConn1
  Ideal Switch4/RConn1 -- Three-Phase Breaker3/RConn2
  Ideal Switch4/LConn1 -- measurement3/RConn2
  Ideal Switch5/RConn1 -- Three-Phase Breaker3/RConn1
  Ideal Switch5/LConn1 -- measurement3/RConn3
